simulink model "test_sys_MHE"  (R2022b)
settings: Solver=FixedStepDiscrete  StartTime=0.0  StopTime=T_final  FixedStep=T_sample  RelTol=1e-3
values from neighbouring files (symbols this model uses):
  A = [0.995 0.0998 ... (first row only)    [Run_model.m]
  B = [0.1; 0.1]    [Run_model.m]
  C = [0.571052826934  0.00320705121121; 0.105905694945  0.429437411805; 0.715489520193  0.338935563141; 0.31761476712  0.78571602684; 0.688586017165  0.771120435927; 0.876557849311  0.658449257994]    [C.mat]    (also in Run_model.m = load('C.mat').C)
  D = zeros(n_meas,n_int)    [Run_model.m]
  indicator = zeros(n_meas,1)    [Run_model.m]
  L = 5    [Run_model.m]
  n_alpha = size(HL_u,2)    [Get_DDL1_MHE_Param.m]    (also in Get_DDL2_MHE_Param.m; Get_L1MHE_Param.m; Get_MHE_Param.m; Run_model.m)
  n_meas = 6    [Run_model.m]
  P = 1    [Run_model.m]
  R = 10    [Run_model.m]
  rho = 1    [Run_model.m]
  T_sample = 0.01    [Run_model.m]    (also in plot_error_table.m)
  T_start_attack = .1*T_final    (= 0.8)    [Run_model.m]
  T_start_opt = T_sample*(L+1)    (= 0.06)    [Run_model.m]
  U0 = zeros(n_int,L)    [Run_model.m]
  U0_MD = zeros(n_int,L+1)    [Run_model.m]
  u_d = u_traj(1:N_samples,:)    [Run_model.m]
  x0 = 7*ones(n_states,1)    [Run_model.m]
  X0_hat = zeros(L*n_states,1)    [Run_model.m]
  x0_hat = z_hat(1:n_states)    [FIE_MDL1.m]    (also in FIE_MDL2.m = z_hat(1:n_states,:); Run_model.m = [1; 2]; mhe_MDL1.m; mhe_MDL2.m = z_hat(1:n_states,:))
  x_d = x_traj(1:N_samples,:)    [Run_model.m]
  Y0 = zeros(n_meas,L)    [Run_model.m]
  y_d = y_traj(1:N_samples,:)    [Run_model.m]
undefined symbols (not defined in the file or in its folder): Aeq_DDL1, Aeq_DDL2, Aeq_MDL1, Aeq_MDL2, f_DDL1, f_DDL2, F_MDL1, f_MDL1, F_MDL2, f_MDL2, H1_MDL1, H1_MDL2, H_DDL2, H_L1_DDL1, H_L1_MDL1, H_L2_DDL1, H_L2_MDL1, H_MDL2, n_int, n_states
libraries: simulink x6
settings Model: Creator=Abelb  LastModifiedBy=Abelb
settings DebuggingCC: UnconnectedInputMsg=warning  UnconnectedOutputMsg=warning  UnconnectedLineMsg=warning
settings ModelReferenceCC: EnableRefExpFcnMdlSchedulingChecks=on
settings RTWCC: DLArmComputeVersion=19.05

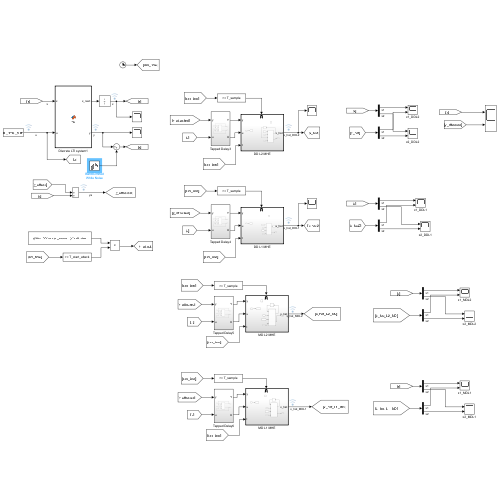
[thumbnail: Simulink's stored preview of the top-level diagram]
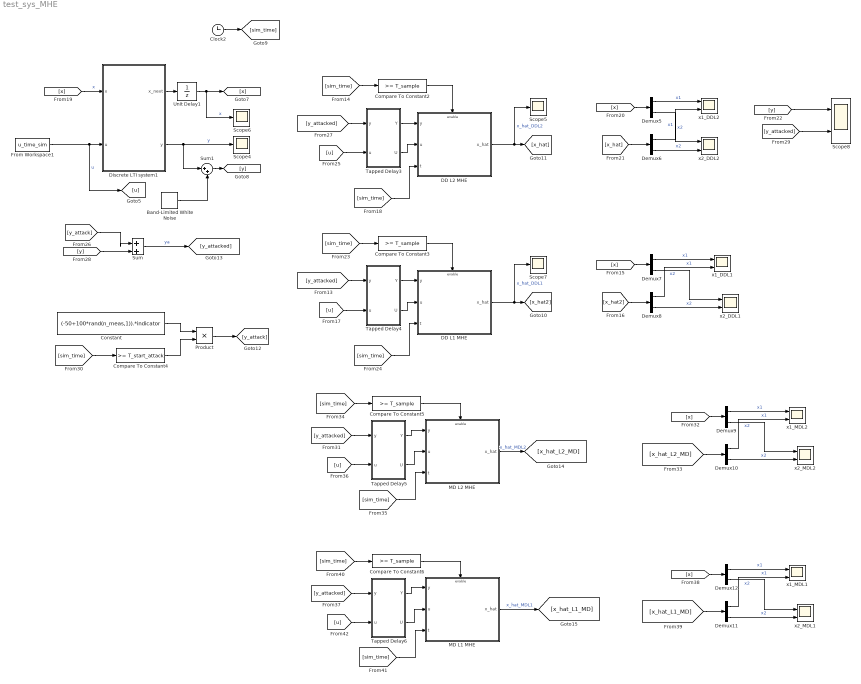
== system test_sys_MHE ==
  Band-Limited White Noise : simulink/Sources/Band-Limited White Noise  Cov=[0.01]  Ts=T_sample  seed=[23341]
  Clock2 : Clock
  Compare To Constant{2..3,5..6} (4 alike) : simulink/Logic and Bit Operations/Compare To Constant  relop=>=  const=T_sample  OutDataTypeStr=boolean
  Compare To Constant4 : simulink/Logic and Bit Operations/Compare To Constant  relop=>=  const=T_start_attack  OutDataTypeStr=boolean
  Constant : Constant  Value=(-50+100*rand(n_meas,1)).*indicator
  DD L1 MHE : Subsystem
  DD L2 MHE : Subsystem
  Demux{5..12} (8 alike) : Demux  Outputs=2
  Discrete LTI system1 : MATLAB Function  TreatAsAtomicUnit=on
  From Workspace1 : FromWorkspace  VariableName=u_time_sim
  MD L1 MHE : Subsystem
  MD L2 MHE : Subsystem
  Product : Product
  Scope{4..7} (4 alike) : Scope
  Scope8 : Scope  NumInputPorts=2
  Sum : Sum  Inputs=|++
  Sum1 : Sum  Inputs=|++
  Tapped Delay3 : Subsystem
  Tapped Delay4 : Subsystem
  Tapped Delay5 : Subsystem
  Tapped Delay6 : Subsystem
  Unit Delay1 : UnitDelay  InitialCondition=x0  SampleTime=-1  HasFrameUpgradeWarning=on
  x1_DDL1 : Scope  NumInputPorts=2
  x1_DDL2 : Scope  NumInputPorts=2
  x1_MDL1 : Scope  NumInputPorts=2
  x1_MDL2 : Scope  NumInputPorts=2
  x2_DDL1 : Scope  NumInputPorts=2
  x2_DDL2 : Scope  NumInputPorts=2
  x2_MDL1 : Scope  NumInputPorts=2
  x2_MDL2 : Scope  NumInputPorts=2
  wires:
  [x] -> Demux7/1
  Demux7/1 -> x1_DDL1/1  "x1"
  Demux8/2 -> x2_DDL1/2  "x2"
  Demux7/2 -> x2_DDL1/1  "x2"
  Compare To Constant3/1 -> DD L1 MHE/Enable
  [x_hat2] -> Demux8/1
  Demux8/1 -> x1_DDL1/2  "x1"
  [y_attacked] -> Tapped Delay4/1(y)
  [sim_time] -> Compare To Constant3/1
  Tapped Delay4/2(U) -> DD L1 MHE/2(u)
  [sim_time] -> DD L2 MHE/3(t)
  Unit Delay1/1 -> Scope6/1, [x]  "x"
  [u] -> Tapped Delay4/2(u)
  Discrete LTI system1/1(x_next) -> Unit Delay1/1
  Discrete LTI system1/2(y) -> Sum1/1, Scope4/1  "y"
  Tapped Delay3/1(Y) -> DD L2 MHE/1(y)
  [x] -> Demux5/1
  [sim_time] -> DD L1 MHE/3(t)
  Compare To Constant2/1 -> DD L2 MHE/Enable
  DD L1 MHE/1(x_hat) -> Scope7/1, [x_hat2]  "x_hat_DDL1"
  Demux5/1 -> x1_DDL2/1  "x1"
  [x] -> Discrete LTI system1/1(x)  "x"
  Tapped Delay4/1(Y) -> DD L1 MHE/1(y)
  Demux6/2 -> x2_DDL2/2  "x2"
  Tapped Delay3/2(U) -> DD L2 MHE/2(u)
  [x_hat] -> Demux6/1
  [y_attacked] -> Tapped Delay3/1(y)
  [sim_time] -> Compare To Constant2/1
  Clock2/1 -> [sim_time]
  [u] -> Tapped Delay3/2(u)
  Demux5/2 -> x2_DDL2/1  "x2"
  From Workspace1/1 -> [u], Discrete LTI system1/2(u)  "u"
  Demux6/1 -> x1_DDL2/2  "x1"
  DD L2 MHE/1(x_hat) -> Scope5/1, [x_hat]  "x_hat_DDL2"
  Sum/1 -> [y_attacked]  "ya"
  [y_attack] -> Sum/1
  [y] -> Sum/2
  [y_attacked] -> Scope8/2
  [y] -> Scope8/1
  [sim_time] -> Compare To Constant4/1
  Product/1 -> [y_attack]
  Constant/1 -> Product/1
  Compare To Constant4/1 -> Product/2
  Sum1/1 -> [y]
  Band-Limited White Noise/1 -> Sum1/2
  [y_attacked] -> Tapped Delay5/1(y)
  [u] -> Tapped Delay5/2(u)
  Compare To Constant5/1 -> MD L2 MHE/Enable
  Tapped Delay5/2(U) -> MD L2 MHE/2(u)
  Tapped Delay5/1(Y) -> MD L2 MHE/1(y)
  MD L2 MHE/1(x_hat) -> [x_hat_L2_MD]  "x_hat_MDL2"
  Demux10/2 -> x2_MDL2/2  "x2"
  Demux10/1 -> x1_MDL2/2  "x1"
  Demux9/2 -> x2_MDL2/1  "x2"
  [x] -> Demux9/1
  Demux9/1 -> x1_MDL2/1  "x1"
  [x_hat_L2_MD] -> Demux10/1
  [sim_time] -> Compare To Constant5/1
  [sim_time] -> MD L2 MHE/3(t)
  [sim_time] -> Compare To Constant6/1
  [sim_time] -> MD L1 MHE/3(t)
  Compare To Constant6/1 -> MD L1 MHE/Enable
  Demux12/1 -> x1_MDL1/1  "x1"
  Demux12/2 -> x2_MDL1/1  "x2"
  [x] -> Demux12/1
  Demux11/1 -> x1_MDL1/2  "x1"
  MD L1 MHE/1(x_hat) -> [x_hat_L1_MD]  "x_hat_MDL1"
  [x_hat_L1_MD] -> Demux11/1
  Tapped Delay6/2(U) -> MD L1 MHE/2(u)
  Tapped Delay6/1(Y) -> MD L1 MHE/1(y)
  [u] -> Tapped Delay6/2(u)
  Demux11/2 -> x2_MDL1/2  "x2"
  [y_attacked] -> Tapped Delay6/1(y)

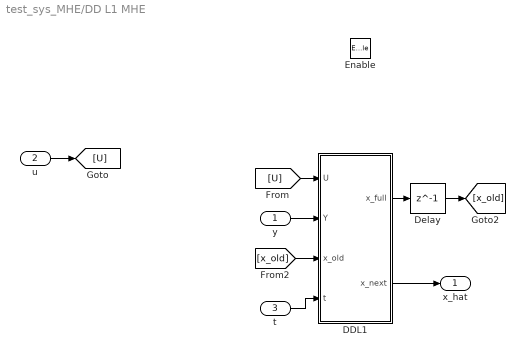
== system test_sys_MHE/DD L1 MHE ==
  y : Inport
  u : Inport  Port=2
  t : Inport  Port=3
  Enable : EnablePort
  DDL1 : MATLAB Function  TreatAsAtomicUnit=on
  Delay : Delay  DelayLength=1  InitialCondition=X0_hat
  x_hat : Outport
  wires:
  u/1 -> [U]
  y/1 -> DDL1/2(Y)
  [U] -> DDL1/1(U)
  DDL1/2(x_next) -> x_hat/1
  t/1 -> DDL1/4(t)
  DDL1/1(x_full) -> Delay/1
  Delay/1 -> [x_old]
  [x_old] -> DDL1/3(x_old)

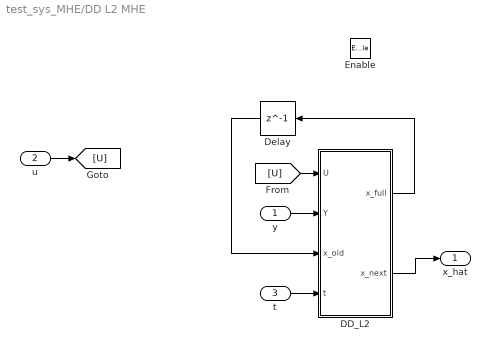
== system test_sys_MHE/DD L2 MHE ==
  y : Inport
  u : Inport  Port=2
  t : Inport  Port=3
  Enable : EnablePort
  DD_L2 : MATLAB Function  TreatAsAtomicUnit=on
  Delay : Delay  DelayLength=1  InitialCondition=X0_hat
  x_hat : Outport
  wires:
  u/1 -> [U]
  y/1 -> DD_L2/2(Y)
  [U] -> DD_L2/1(U)
  DD_L2/2(x_next) -> x_hat/1
  DD_L2/1(x_full) -> Delay/1
  Delay/1 -> DD_L2/3(x_old)
  t/1 -> DD_L2/4(t)

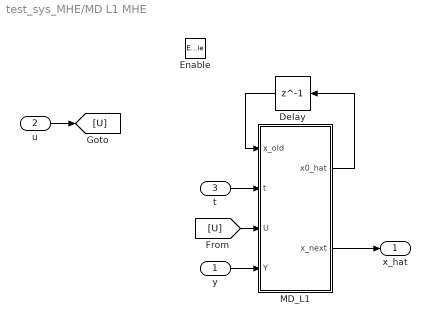
== system test_sys_MHE/MD L1 MHE ==
  y : Inport
  u : Inport  Port=2
  t : Inport  Port=3
  Enable : EnablePort
  Delay : Delay  DelayLength=1  InitialCondition=x0_hat
  MD_L1 : MATLAB Function  TreatAsAtomicUnit=on
  x_hat : Outport
  wires:
  u/1 -> [U]
  y/1 -> MD_L1/4(Y)
  [U] -> MD_L1/3(U)
  MD_L1/2(x_next) -> x_hat/1
  t/1 -> MD_L1/2(t)
  MD_L1/1(x0_hat) -> Delay/1
  Delay/1 -> MD_L1/1(x_old)

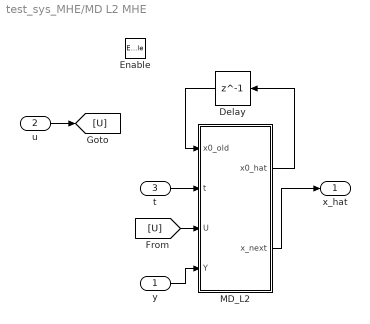
== system test_sys_MHE/MD L2 MHE ==
  y : Inport
  u : Inport  Port=2
  t : Inport  Port=3
  Enable : EnablePort
  Delay : Delay  DelayLength=1  InitialCondition=x0_hat
  MD_L2 : MATLAB Function  TreatAsAtomicUnit=on
  x_hat : Outport
  wires:
  u/1 -> [U]
  y/1 -> MD_L2/4(Y)
  [U] -> MD_L2/3(U)
  MD_L2/2(x_next) -> x_hat/1
  t/1 -> MD_L2/2(t)
  MD_L2/1(x0_hat) -> Delay/1
  Delay/1 -> MD_L2/1(x0_old)

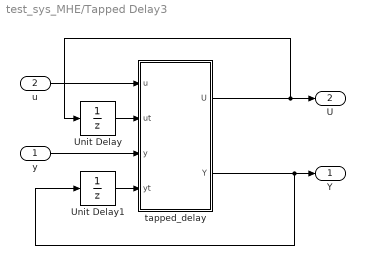
== system test_sys_MHE/Tapped Delay3 ==
  y : Inport
  u : Inport  Port=2
  Unit Delay : UnitDelay  InitialCondition=U0  SampleTime=-1  HasFrameUpgradeWarning=on
  Unit Delay1 : UnitDelay  InitialCondition=Y0  SampleTime=-1  HasFrameUpgradeWarning=on
  tapped_delay : MATLAB Function  TreatAsAtomicUnit=on
  Y : Outport
  U : Outport  Port=2
  wires:
  u/1 -> tapped_delay/1(u)
  y/1 -> tapped_delay/3(y)
  tapped_delay/1(U) -> Unit Delay/1, U/1
  tapped_delay/2(Y) -> Unit Delay1/1, Y/1
  Unit Delay/1 -> tapped_delay/2(ut)
  Unit Delay1/1 -> tapped_delay/4(yt)

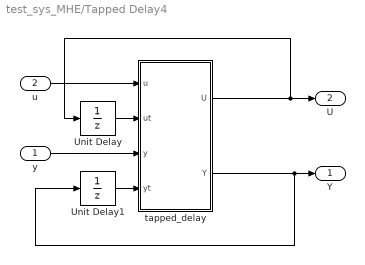
== system test_sys_MHE/Tapped Delay4 ==
  y : Inport
  u : Inport  Port=2
  Unit Delay : UnitDelay  InitialCondition=U0  SampleTime=-1  HasFrameUpgradeWarning=on
  Unit Delay1 : UnitDelay  InitialCondition=Y0  SampleTime=-1  HasFrameUpgradeWarning=on
  tapped_delay : MATLAB Function  TreatAsAtomicUnit=on
  Y : Outport
  U : Outport  Port=2
  wires:
  u/1 -> tapped_delay/1(u)
  y/1 -> tapped_delay/3(y)
  tapped_delay/1(U) -> Unit Delay/1, U/1
  tapped_delay/2(Y) -> Unit Delay1/1, Y/1
  Unit Delay/1 -> tapped_delay/2(ut)
  Unit Delay1/1 -> tapped_delay/4(yt)

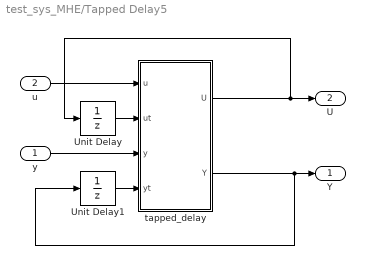
== system test_sys_MHE/Tapped Delay5 ==
  y : Inport
  u : Inport  Port=2
  Unit Delay : UnitDelay  InitialCondition=U0_MD  SampleTime=-1  HasFrameUpgradeWarning=on
  Unit Delay1 : UnitDelay  InitialCondition=Y0  SampleTime=-1  HasFrameUpgradeWarning=on
  tapped_delay : MATLAB Function  TreatAsAtomicUnit=on
  Y : Outport
  U : Outport  Port=2
  wires:
  u/1 -> tapped_delay/1(u)
  y/1 -> tapped_delay/3(y)
  tapped_delay/1(U) -> Unit Delay/1, U/1
  tapped_delay/2(Y) -> Unit Delay1/1, Y/1
  Unit Delay/1 -> tapped_delay/2(ut)
  Unit Delay1/1 -> tapped_delay/4(yt)

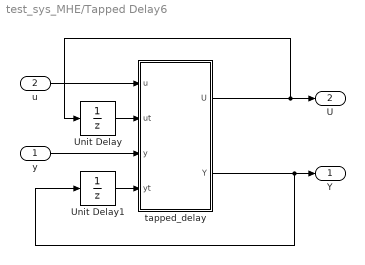
== system test_sys_MHE/Tapped Delay6 ==
  y : Inport
  u : Inport  Port=2
  Unit Delay : UnitDelay  InitialCondition=U0_MD  SampleTime=-1  HasFrameUpgradeWarning=on
  Unit Delay1 : UnitDelay  InitialCondition=Y0  SampleTime=-1  HasFrameUpgradeWarning=on
  tapped_delay : MATLAB Function  TreatAsAtomicUnit=on
  Y : Outport
  U : Outport  Port=2
  wires:
  u/1 -> tapped_delay/1(u)
  y/1 -> tapped_delay/3(y)
  tapped_delay/1(U) -> Unit Delay/1, U/1
  tapped_delay/2(Y) -> Unit Delay1/1, Y/1
  Unit Delay/1 -> tapped_delay/2(ut)
  Unit Delay1/1 -> tapped_delay/4(yt)

== matlab function test_sys_MHE/Discrete LTI system1 ==
  data: x input; x_next output; u input; y output; A parameter; C parameter; B parameter; D parameter
function [x_next,y] = fcn(x,u,A,C,B,D)
% Discrete state-space model for system

x_next = A*x + B*u;

y = C*x + D*u;

== matlab function test_sys_MHE/Tapped Delay3/tapped_delay ==
  data: u input; U output; ut input; y input; yt input; Y output
function [U,Y] = fcn(u,ut,y,yt)
%% tapped_delay_array
% shift columns from tapped matrix to the left and appends most recent
% vector to the last column
%%% input
ut(:,1:end-1) = ut(:,2:end);
ut(:,end) = u;
U = ut;
%%% output
yt(:,1:end-1) = yt(:,2:end);
yt(:,end) = y;
Y = yt;

== matlab function test_sys_MHE/Tapped Delay4/tapped_delay ==
  data: u input; U output; ut input; y input; yt input; Y output
function [U,Y] = fcn(u,ut,y,yt)
%% tapped_delay_array
% shift columns from tapped matrix to the left and appends most recent
% vector to the last column
%%% input
ut(:,1:end-1) = ut(:,2:end);
ut(:,end) = u;
U = ut;
%%% output
yt(:,1:end-1) = yt(:,2:end);
yt(:,end) = y;
Y = yt;

== matlab function test_sys_MHE/MD L2 MHE/MD_L2 ==
  data: x0_hat output; x0_old input; t input; x_next output; U input; Y input; H_MDL2 parameter; f_MDL2 parameter; Aeq_MDL2 parameter; H1_MDL2 parameter; F_MDL2 parameter; n_states parameter; T_sample parameter; T_start_opt parameter; A parameter; B parameter; C parameter; L parameter; n_int parameter; n_meas parameter; P parameter; R parameter; rho parameter
function [x0_hat,x_next] = fcn(x0_old,t,U,Y, H_MDL2,f_MDL2,Aeq_MDL2,H1_MDL2,F_MDL2, n_states,T_sample, T_start_opt, A, B, C,L, n_int, n_meas,P, R,rho)                                 % MD L2  

coder.extrinsic('mhe_MDL2');
coder.extrinsic('FIE_MDL2');
%% MD L2
%% function [x_next,r]  = fcn(U,Y, Ly, Lu,H0_perp, H1)   
% vectorized
U = U.';
u_local = U(1:end-1);
u = u_local(:);
y = Y(:);

x0_hat = zeros(n_states,1);
x_next = zeros(n_states,1);

if t < T_start_opt 
   % Full information oberver
    t_sample = round(t/T_sample);

    u = u(1:t_sample*n_int);
    y = y(1:t_sample*n_meas);

    [x0_hat(:), x_next(:)] = FIE_MDL2(x0_old,A,B,C,P,R,rho,n_states,n_meas,t_sample,u,y);
    
else 
 % Moving-horizon oberver
    beq = y-H1_MDL2*u;
    [x0_hat(:), x_next(:)] = mhe_MDL2(u,x0_old,beq,Aeq_MDL2,H_MDL2,f_MDL2,n_states,F_MDL2,A,L);
end

== matlab function test_sys_MHE/Tapped Delay5/tapped_delay ==
  data: u input; U output; ut input; y input; yt input; Y output
function [U,Y] = fcn(u,ut,y,yt)
%% tapped_delay_array
% shift columns from tapped matrix to the left and appends most recent
% vector to the last column
%%% input
ut(1:end-1) = ut(2:end);
ut(end) = u;
U = ut;
%%% output
yt(:,1:end-1) = yt(:,2:end);
yt(:,end) = y;
Y = yt;

== matlab function test_sys_MHE/MD L1 MHE/MD_L1 ==
  data: x0_hat output; x_old input; t input; x_next output; U input; Y input; H_L1_MDL1 parameter; H_L2_MDL1 parameter; f_MDL1 parameter; Aeq_MDL1 parameter; F_MDL1 parameter; H1_MDL1 parameter; n_states parameter; T_sample parameter; T_start_opt parameter; A parameter; B parameter; C parameter; L parameter; n_int parameter; n_meas parameter; P parameter; R parameter; rho parameter
function [x0_hat,x_next] = fcn(x_old,t,U,Y, H_L1_MDL1,H_L2_MDL1,f_MDL1,Aeq_MDL1,F_MDL1,H1_MDL1, n_states,T_sample, T_start_opt, A, B, C,L,n_int, n_meas,P, R,rho)                                 % MD L2  

coder.extrinsic('mhe_MDL1');
coder.extrinsic('FIE_MDL1');
%% MD L2
%% function [x_next,r]  = fcn(U,Y, Ly, Lu,H0_perp, H1)   
% vectorized
U = U.';
u_local = U(1:end-1);
u = u_local(:);
y = Y(:);

x0_hat = zeros(n_states,1);
x_next = zeros(n_states,1);

if t < T_start_opt 
   % Full information oberver
    t_sample = round(t/T_sample);

    u = u(1:t_sample*n_int);
    y = y(1:t_sample*n_meas);

    [x0_hat(:), x_next(:)] = FIE_MDL1(x_old,A,B,C,P,R,rho,n_states,n_meas,t_sample,u,y);
    
else 
 % Moving-horizon oberver
    beq = y-H1_MDL1*u;
    [x0_hat(:), x_next(:)] = mhe_MDL1(u,x_old,beq,Aeq_MDL1,H_L1_MDL1,H_L2_MDL1,f_MDL1,F_MDL1,A,n_states,L);
end

== matlab function test_sys_MHE/Tapped Delay6/tapped_delay ==
  data: u input; U output; ut input; y input; yt input; Y output
function [U,Y] = fcn(u,ut,y,yt)
%% tapped_delay_array
% shift columns from tapped matrix to the left and appends most recent
% vector to the last column
%%% input
ut(1:end-1) = ut(2:end);
ut(end) = u;
U = ut;
%%% output
yt(:,1:end-1) = yt(:,2:end);
yt(:,end) = y;
Y = yt;

== matlab function test_sys_MHE/DD L1 MHE/DDL1 ==
  data: x_full output; x_next output; U input; Y input; x_old input; t input; L parameter; H_L1_DDL1 parameter; H_L2_DDL1 parameter; f_DDL1 parameter; Aeq_DDL1 parameter; n_meas parameter; n_int parameter; n_states parameter; n_alpha parameter; rho parameter; P parameter; R parameter; u_d parameter; x_d parameter; y_d parameter; T_start_opt parameter; T_sample parameter
function [x_full,x_next]   = fcn(U,Y,x_old,t,L,H_L1_DDL1,H_L2_DDL1, f_DDL1, Aeq_DDL1, n_meas, n_int,n_states,n_alpha,rho, P, R, u_d,x_d, y_d,T_start_opt,T_sample)          
%% DD L2
%% function [x_next,r]  = fcn(U,Y, Aeq,n_states,E_MH,T, DE_MH, n_alpha, CE_MH)
coder.extrinsic('mhe_DDL1');
coder.extrinsic('FIE_DDL1');

% vectorized
% U = U.';   % if input dimention is 1, do this operation, otherwise, comment this line
% u_local = U(:,2:end);
u = U(:);
y = Y(:);

x_full = zeros(n_states*L,1);
% z_full = zeros(n_alpha+n_states*L + n_meas*L,1);
x_next = zeros(n_states,1);

if t < T_start_opt 
   % Full information oberver
    t_sample = round(t/T_sample);

    u = u(1:t_sample*n_int);
    y = y(1:t_sample*n_meas);
    x0_old = x_full(1:n_states,:);

    x_full(:) = FIE_DDL1(x0_old,u_d,x_d,y_d,P,R,rho,L,n_states,n_meas,t_sample,u,y);

    x_next(:) = x_full(n_states*(t_sample-1)+1:n_states*t_sample,:);
else
   % Moving-horizon oberver
    beq = [u;y;zeros(n_states*L,1)];
    x_full(:) = mhe_DDL1(x_old,beq,Aeq_DDL1,H_L1_DDL1,H_L2_DDL1,f_DDL1,n_states,n_meas,L);
    x_next(:) = x_full(end-n_states+1:end,:);
end
% x_next(:) = x_full(1:n_states,:);

== matlab function test_sys_MHE/DD L2 MHE/DD_L2 ==
  data: x_full output; x_next output; U input; Y input; x_old input; t input; L parameter; H_DDL2 parameter; f_DDL2 parameter; Aeq_DDL2 parameter; n_meas parameter; n_int parameter; n_states parameter; rho parameter; P parameter; R parameter; u_d parameter; x_d parameter; y_d parameter; T_start_opt parameter; T_sample parameter
function [x_full,x_next]   = fcn(U,Y,x_old,t,L,H_DDL2, f_DDL2, Aeq_DDL2, n_meas, n_int,n_states,rho, P, R, u_d,x_d, y_d,T_start_opt,T_sample)          
%% DD L2
%% function [x_next,r]  = fcn(U,Y, Aeq,n_states,E_MH,T, DE_MH, n_alpha, CE_MH)
coder.extrinsic('mhe_DDL2');
coder.extrinsic('FIE_DDL2');

% vectorized
% U = U.';   % if input dimention is 1, do this operation, otherwise, comment this line
% u_local = U(:,2:end);
u = U(:);
y = Y(:);

x_full = zeros(n_states*L,1);
x_next = zeros(n_states,1);

if t < T_start_opt 
   % Full information oberver
    t_sample = round(t/T_sample);

    u = u(1:t_sample*n_int);
    y = y(1:t_sample*n_meas);
    x0_old = x_full(1:n_states,:);

    x_full(:) = FIE_DDL2(x0_old,u_d,x_d,y_d,P,R,rho,L,n_states,n_meas,t_sample,u,y);

    x_next(:) = x_full(n_states*(t_sample-1)+1:n_states*t_sample,:);
else
   % Moving-horizon oberver
    beq = [u;y;zeros(n_states*L,1)];
    x_full(:) = mhe_DDL2(x_old,beq,Aeq_DDL2,H_DDL2,f_DDL2,n_states,n_meas,L);
    x_next(:) = x_full(end-n_states+1:end,:);
end
% x_next(:) = x_full(1:n_states,:);
